simulink model "Triciclo"  (R2025b)
settings: Solver=VariableStepAuto  StartTime=0.0  StopTime=10  RelTol=1e-3
settings Model: Creator=chenfu  LastModifiedBy=chenfu

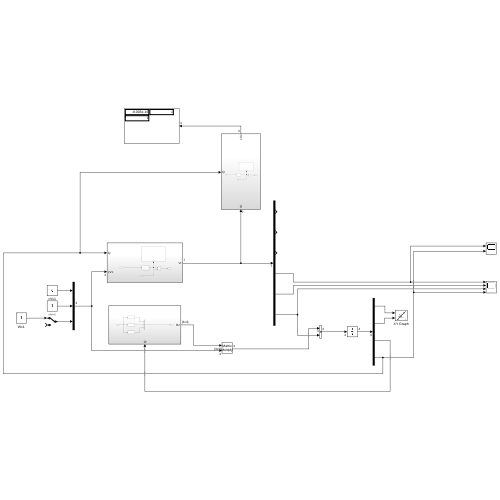
[thumbnail: Simulink's stored preview of the top-level diagram]
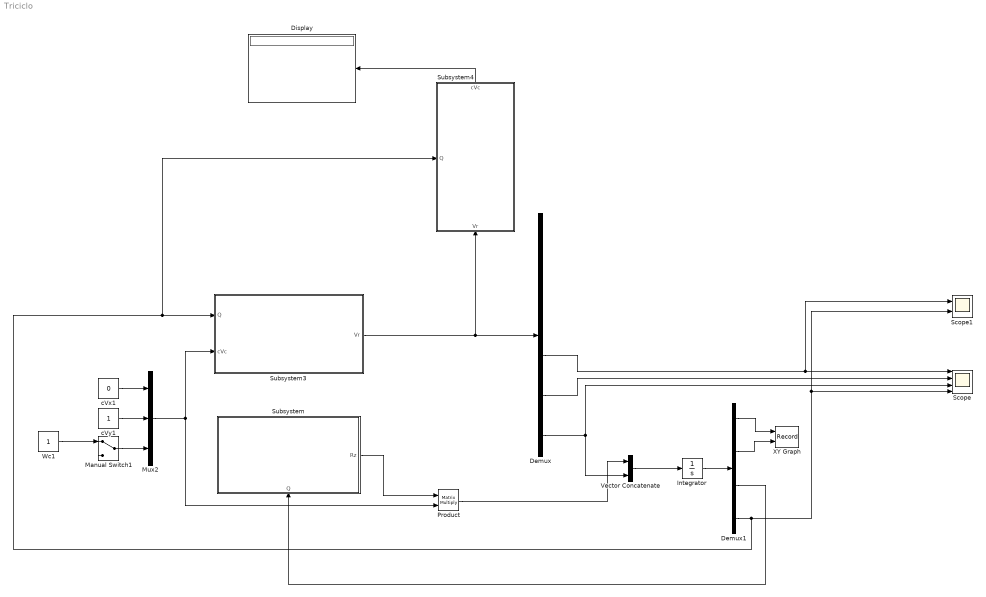
== system Triciclo ==
  Demux : Demux  Outputs=6
  Demux1 : Demux
  Display : Display
  Integrator : Integrator
  Manual Switch1 : ManualSwitch
  Mux2 : Mux  Inputs=3
  Product : Product  Multiplication=Matrix(*)
  Scope : Scope  NumInputPorts=4
      settings: ActiveDisplayYMinimum=-23.774847592235595  ActiveDisplayYMaximum=3.7527608435817323
  Scope1 : Scope  NumInputPorts=2
      settings: ActiveDisplayYMinimum=-1  ActiveDisplayYMaximum=1
  Subsystem : Subsystem
      settings: PortSchema="{\"entries\":[{\"content\":{\"sides\":[{\"content\":{},\"type\":\"ConnectorPlacement.EquallySpacedRectSide\",\"uuid\":\"b42bb782-889e-4dc3-8f9e-e14de7172aa1\"},{\"content\":{\"connectorIds\":[\"Out1\"],\"side\":\"RIGHT\"},\"type\":\"ConnectorPlacement.EquallySpacedRectSide\",\"uuid\":\"b7bb92f1-a68e-4319-bc55-ea9e4bc60d8e\"},{\"content\":{\"side\":\"TOP\"},\"type\":\"ConnectorPlacement.EquallySpacedRectSide\",\"uuid\":\"7cdeca09-1280-458d-8004-1053907d8793\"},{\"content\":{\"connectorIds\":[\"In1\"],\"side\":\"BOTTOM\"},\"type\":\"ConnectorPlacement.EquallySpacedRectSide\",\"uuid\":\"de11f458-efc8-4ba5-9a9d-d22d601f3381\"}]},\"type\":\"ConnectorPlacement.EquallySpacedConnector\",\"uuid\":\"a088bb29-9081-40e8-b619-24ab2822dcef\"}],\"packageUris\":[\"http://schema.mathworks.com/mf0/Connector/R2020b\"],\"version\":\"1.0\"}"
  Subsystem3 : Subsystem
  Subsystem4 : Subsystem
      settings: PortSchema="{\"entries\":[{\"content\":{\"sides\":[{\"content\":{\"connectorIds\":[\"In1\"]},\"type\":\"ConnectorPlacement.EquallySpacedRectSide\",\"uuid\":\"bfc6dda2-980b-486f-8f4a-13f5ae28b8bc\"},{\"content\":{\"connectorIds\":[\"Out1\"],\"side\":\"RIGHT\"},\"type\":\"ConnectorPlacement.EquallySpacedRectSide\",\"uuid\":\"9f81133d-151e-4d55-9db3-98bb733ba25d\"},{\"content\":{\"connectorIds\":[\"In2\"],\"side\":\"TOP\"},\"type\":\"ConnectorPlacement.EquallySpacedRectSide\",\"uuid\":\"106da46a-9bc2-4f9e-8a6c-2d962a357420\"}]},\"type\":\"ConnectorPlacement.EquallySpacedConnector\",\"uuid\":\"5434d69a-f702-4bb5-924f-efdf2ff92e3a\"}],\"packageUris\":[\"http://schema.mathworks.com/mf0/Connector/R2020b\"],\"version\":\"1.0\"}"
  Vector Concatenate : Concatenate
  Wc1 : Constant
  XY Graph : Record  NumPorts=2.0  FileSettingsInternal="{\"entries\":[{\"content\":{\"excelSettings\":{\"content\":{},\"type\":\"Streamout.ExcelSettings\"},\"parquetSettings\":{\"content\":{},\"type\":\"Streamout.ParquetSettings\"}},\"type\":\"Streamout.FileSettingStorage\",\"uuid\":\"\"}],\"packageUris\":[\"http:\\/\\/schema.mathworks.com\\/mf0\\/streamout_blocks\\/R2020a\"],\"version\":\"1.0\"}"  FrameSettings=[0, 0]  Layout=[1 1]  SignalsInternal="{\"entries\":[{\"content\":{\"signals\":[{\"content\":{\"blockPath\":[],\"dimensions\":[1],\"domain\":\"\",\"lineColor\":\"#a2142f\",\"plots\":[ 1 ],\"port\":1,\"sid\":[\"\"],\"signalID\":1,\"signalName\":\"Demux1:1\"},\"type\":\"RecordBlkView.Signal\",\"uuid\":\"\"},{\"content\":{\"blockPath\":[],\"dimensions\":[1],\"domain\":\"\",\"lineColor\":\"#139fff\",\"plots\":[ 1 ],\"port\":2,\"sid\":[\"\"],\"signalID\":2,\"signalName\":\"Demux1:2\"},\"type\":\"RecordBlkView.Signal\",\"uuid\":\"\"}]},\"type\":\"RecordBlkView.InputSignals\",\"uuid\":\"\"}],\"packageUris\":[\"http:\\/\\/schema.mathworks.com\\/mf0\\/streamout_blocks\\/R2020a\"],\"version\":\"1.0\"}"  VisualizationBindings="{\"xyplotplugin\":{\"info\":[{\"series\":[{\"bindingParametersList\":[{\"parameter\":\"X-Axis\",\"signalID\":1,\"signalName\":\"Demux1:1\"},{\"parameter\":\"Y-Axis\",\"signalID\":2,\"signalName\":\"Demux1:2\"}],\"seriesID\":0}],\"subplotID\":1}]}}"  CompatibilityTag=XY
  cVx1 : Constant  Value=0
  cVy1 : Constant
  wires:
  Manual Switch1/1 -> Mux2/3
  Wc1/1 -> Manual Switch1/1
  cVx1/1 -> Mux2/1
  cVy1/1 -> Mux2/2
  Mux2/1 -> Product/2, Subsystem3/2(cVc)
  Subsystem3/1(Vr) -> Demux/1, Subsystem4/1(Vr)
  Subsystem/1(Rz) -> Product/1
  Demux/6 -> Vector Concatenate/2, Scope/3
  Product/1 -> Vector Concatenate/1
  Vector Concatenate/1 -> Integrator/1
  Integrator/1 -> Demux1/1
  Demux1/4 -> Subsystem4/2(Q), Subsystem3/1(Q), Scope/4, Scope1/2
  Demux1/3 -> Subsystem/1(Q)
  Demux1/1 -> XY Graph/1
  Demux1/2 -> XY Graph/2
  Demux/4 -> Scope1/1, Scope/1
  Demux/5 -> Scope/2
  Subsystem4/1(cVc) -> Display/1

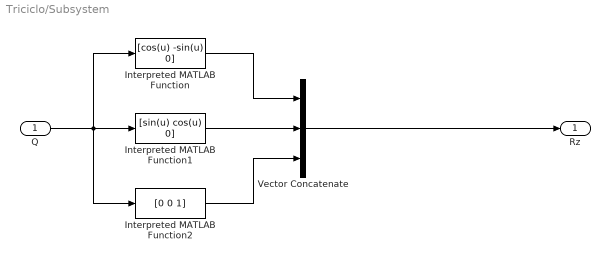
== system Triciclo/Subsystem ==
  Q : Inport
  Interpreted MATLAB Function : MATLABFcn  MATLABFcn=[cos(u) -sin(u) 0]
  Interpreted MATLAB Function1 : MATLABFcn  MATLABFcn=[sin(u) cos(u) 0]
  Interpreted MATLAB Function2 : MATLABFcn  MATLABFcn=[0 0 1]
  Vector Concatenate : Concatenate  NumInputs=3  Mode=Multidimensional array  ConcatenateDimension=2
  Rz : Outport
  wires:
  Interpreted MATLAB Function/1 -> Vector Concatenate/1
  Interpreted MATLAB Function2/1 -> Vector Concatenate/3
  Interpreted MATLAB Function1/1 -> Vector Concatenate/2
  Q/1 -> Interpreted MATLAB Function/1, Interpreted MATLAB Function1/1, Interpreted MATLAB Function2/1
  Vector Concatenate/1 -> Rz/1

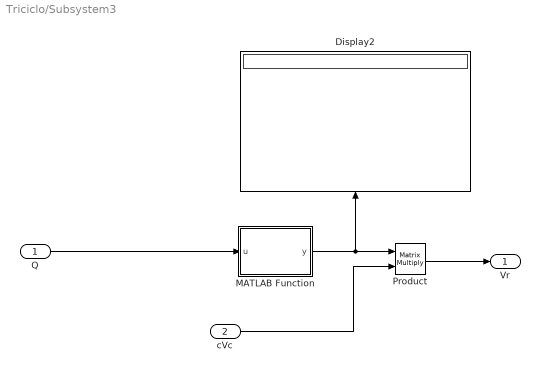
== system Triciclo/Subsystem3 ==
  Q : Inport
  cVc : Inport  Port=2
  Display2 : Display
  MATLAB Function : MATLAB Function  TreatAsAtomicUnit=on
  Product : Product  Multiplication=Matrix(*)
  Vr : Outport
  wires:
  MATLAB Function/1(y) -> Product/1, Display2/1
  Product/1 -> Vr/1
  cVc/1 -> Product/2
  Q/1 -> MATLAB Function/1(u)

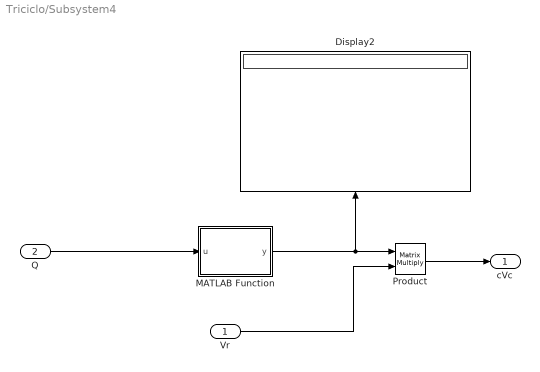
== system Triciclo/Subsystem4 ==
  Vr : Inport
  Q : Inport  Port=2
  Display2 : Display
  MATLAB Function : MATLAB Function  TreatAsAtomicUnit=on
  Product : Product  Multiplication=Matrix(*)
  cVc : Outport
  wires:
  MATLAB Function/1(y) -> Product/1, Display2/1
  Product/1 -> cVc/1
  Vr/1 -> Product/2
  Q/1 -> MATLAB Function/1(u)

== matlab function Triciclo/Subsystem3/MATLAB Function ==
  data: u input; y output
function y = fcn(u)

y = IK(u);

== matlab function Triciclo/Subsystem4/MATLAB Function ==
  data: u input; y output
function y = fcn(u)

y = DK(u);
